simulink model "DrivetrainHevP4_SSC"  (R2021a)
settings: Solver=ode23t  StartTime=0.0  StopTime=10.0  RelTol=1e-3
model workspace (MAT data in the model file):
  Aeff = 0.0314159265359
  Af = 2.27
  Apist_C0 = 0.0314159265359
  Apist_TCC = 0.001
  Bx = 10
  Cd = 0.25
  CoulFr_ShaftIn = 0
  Cx = 1.9
  DensAir = 1.293
  DerFac_C0 = 1
  DerFac_TCC = 1
  Drag_C0 = 0
  Drag_TCC = 0
  Dx = 1
  Eff_Diff = [0.98 0.98]
  Ex = 0.97
  FDrive = 3.32
  FDrive_P4 = 4.1
  FZMAX = 6570
  FZMIN = 0
  G = [0 1 2 3 4 5 6]
  G_o = 1
  Iyy = 0.8
  Iyy_Whl = 0.8
  JCa_Diff = 0.001
  JEng = 0.01
  JMot = 0.21
  JPl_Diff = 0.001
  JShIn = 1e-05
  JShOut = 0.15
  Jd = 0.025
  Ji = 0.21
  Jin_Cltch = 0.2
  Jout = [0.009 0.01 0.01 0.01 0.01 0.01 0.01]
  Jout_Cltch = 0.01
  Jt = 0.01
  Jw1 = 0.01
  Jw2 = 0.01
  K_c = 10000
  KinFr_C0 = 0.4
  KinFr_TCC = 0.3
  Lrel = 0.15
  Mass = 1623
  N = [0.001 4.212 2.637 1.8 1.386 1 0.772]
  NF = 2
  NR = 2
  N_P0 = 3
  Ndiff = 3.32
  Ndiff_P4 = 4.1
  Ndisk = 1
  Neff_C0 = 1
  Neff_TCC = 6
  PEng_C0 = 30000
  PEng_TCC = 100
  Pabs = 101325
  Press = 300000
  PwrThr_Diff = [0.001 0.001]
  RatFr_ShaftIn = 1.1
  Re = 0.327
  Reff = 0.11
  Reff_C0 = 0.11
  Reff_TCC = 130
  Rm = 0.15
  SprStff_ShaftIn = 10000
  StatFr_C0 = 0.45
  StatFr_TCC = 0.35
  T = 273
  Temp_bpts = [313 358]
  Trq_bpts = [25 50 75 100 150 200 250]
  UNLOADED_RADIUS = 0.336
  VXLOW = 2
  VisFr_Diff = [0.001 0.001]
  ViscFr_ShaftIn = 400
  aMy = 0.01
  a_CG = 1.09
  alphaMy = 0
  b : Simulink.Parameter (value not decoded)
  bMy = 0
  b_CG = 1.7
  bd = 0.001
  betaMy = 1
  bi = 0.001
  bin_Cltch = 0.003
  bout = [0.003 0.003 0.003 0.003 0.003 0.003 0.003]
  bout_Cltch = 0.003
  br = 0.001
  bt = 0.001
  bw1 = 0.001
  bw2 = 0.001
  cGain = 100000
  cMy = 0
  disk_abore = 0.05
  domega_o = 0
  eta = [0.95 0.95 0.95 0.95 0.95 0.95 0.95]
  eta_diff = 0.98
  eta_tbl = [1 1 1 1 1 1 1 1 1 1 1 1 ... (1078 elements, 7x11x7x2)]
  g = 9.81
  h = 0.5
  k : Simulink.Parameter (value not decoded)
  kappamax = 1.5
  ki_c = 100000
  lam_x = 1
  mu_kinetic = 0.35
  mu_static = 0.45
  muk = 0.4
  mus = 0.45
  num_pads = 2
  omega_bpts = [500.383141081 749.619781963 1002.67614148 1250.9578527 1499.23956393 1747.52127515 1995.80298637 2501.9157054 2998.47912785 4001.15526933 5003.83141081]
  omega_c : Simulink.Parameter (value not decoded)
  omega_o = 0
  omegai_o = 0
  omegal = 94.2477796077
  omegao = 0
  omegat_o = 0
  omegau = 83.7758040957
  omegaw1o = 0
  omegaw2o = 0
  p0 = 10000000
  phi = [0 0.5 0.6 0.7 0.8 0.87 0.92 0.94 0.96 0.97]
  phi_new = [0 0.5 0.6 0.7 0.8 0.87 0.92 0.94 0.96 0.97 0.99 1.02 ... (16 elements, 1x16)]
  philu = 0.85
  press = 700000
  psi = [12.2938 12.8588 13.1452 13.6285 14.6163 16.2675 19.3503 22.1046 29.9986 50]
  psi_new = [12.2938 12.8588 13.1452 13.6285 14.6163 16.2675 19.3503 22.1046 29.9986 50 48 41.76 ... (16 elements, 1x16)]
  tauC = 0.25
  tauTC = 0.1
  tau_s = 0.1
  theta_o = 0
  wc = 10
  win_o = 0
  wout_o = 0
  x_o = 0
  xdot_o = 0
  zeta = [2.232 1.5462 1.4058 1.2746 1.1528 1.0732 1.0192 0.9983 0.9983 0.9983]
  zeta_new = [2.232 1.5462 1.4058 1.2746 1.1528 1.0732 1.0192 0.9983 0.9983 0.9983 0.979797979798 1.04382929642 ... (16 elements, 1x16)]
libraries: fl_lib x28, sdl_lib x23, nesl_utility x21, simulink x6
(part 2 of 2)

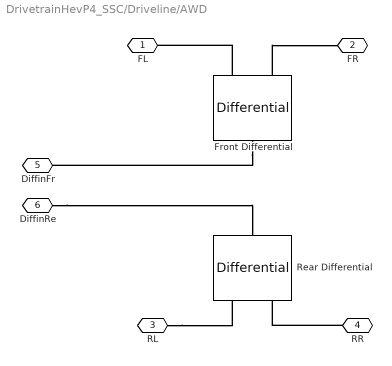
== system DrivetrainHevP4_SSC/Driveline/AWD ==
  Front Differential : sdl_lib/Gears/Differential  driveshaft_location=2  cd_ratio=FDrive  friction_model=2  mu_visc=VisFr_Diff N*m/(rad/s)  efficiency=Eff_Diff  temperature_TLU=[ 280 300 320 ] K  efficiency_ss_TLU=[ 0.95 0.9 0.85 ]  efficiency_cd_TLU=[ 0.95 0.9 0.85 ]  pwr_thr=PwrThr_Diff W  thermal_mass=50 J/K  T_init=300 K  model_inertia=1  carrier_inertia=JCa_Diff kg*m^2  planet_inertia=JPl_Diff kg*m^2
      settings: SourceProductBaseCode=LD
  Rear Differential : sdl_lib/Gears/Differential  driveshaft_location=sdl.enum.differential_orientation.right  cd_ratio=FDrive_P4  friction_model=sdl.enum.gear_friction.constant  mu_visc=VisFr_Diff N*m/(rad/s)  efficiency=Eff_Diff  temperature_TLU=[ 280 300 320 ] K  efficiency_ss_TLU=[ 0.95 0.9 0.85 ]  efficiency_cd_TLU=[ 0.95 0.9 0.85 ]  pwr_thr=PwrThr_Diff W  thermal_mass=50 J/K  T_init=300 K  model_inertia=simscape.enum.onoff.on  carrier_inertia=JCa_Diff kg*m^2  planet_inertia=JPl_Diff kg*m^2
      settings: SourceProductBaseCode=LD
  FL : PMIOPort  Side=Left
  FR : PMIOPort  Port=2  Side=Right
  RL : PMIOPort  Port=3  Side=Left
  RR : PMIOPort  Port=4  Side=Right
  DiffinFr : PMIOPort  Port=5  Side=Left
  DiffinRe : PMIOPort  Port=6  Side=Right
  connections:
  Front Differential/LConn1 -- DiffinFr/RConn1
  Front Differential/RConn1 -- FL/RConn1
  RR/RConn1 -- Rear Differential/RConn2
  RL/RConn1 -- Rear Differential/RConn1
  Front Differential/RConn2 -- FR/RConn1
  DiffinRe/RConn1 -- Rear Differential/LConn1

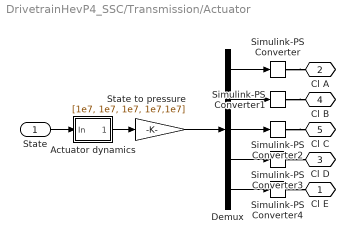
== system DrivetrainHevP4_SSC/Transmission/Actuator ==
  State : Inport
  Actuator dynamics : Subsystem  mask(First-order lag supporting vector signals){b=[1 1 1 1 1]*0.01, x_initial=1}
      mask prompts: b "Filter time constant"; x_initial "Initial output"
      mask help: Models a lag of the form 1/(b*s+1) where s is the Laplace operator.
  Demux : Demux  Outputs=5
  Simulink-PS Converter{,1..4} (5 alike) : nesl_utility/Simulink-PS Converter  PhysicalDomain=network_engine_domain  SubClassName=ps_input  LeftPortType=input  RightPortType=output  PseudoPeriodic=off  Frequencies=[]  NoiseDistribution=none  NoiseParameters=[]  Unit=1  AffineConversion=off  FilteringAndDerivatives=zero  SimscapeFilterOrder=1  InputFilterTimeConstant=0.001  UdotUserProvided=1
      settings: SourceProductBaseCode=PW,SS
  State to pressure : Gain  Gain=[1e7, 1e7, 1e7, 1e7,1e7]
  Cl E : PMIOPort  Side=Right
  Cl A : PMIOPort  Port=2  Side=Right
  Cl D : PMIOPort  Port=3  Side=Right
  Cl B : PMIOPort  Port=4  Side=Right
  Cl C : PMIOPort  Port=5  Side=Right
  wires:
  Demux/3 -> Simulink-PS Converter2/1
  Demux/5 -> Simulink-PS Converter4/1
  State to pressure/1 -> Demux/1
  Demux/4 -> Simulink-PS Converter3/1
  Demux/2 -> Simulink-PS Converter1/1
  Demux/1 -> Simulink-PS Converter/1
  Actuator dynamics/1(Out) -> State to pressure/1
  State/1 -> Actuator dynamics/1(In)
  connections:
  Simulink-PS Converter4/RConn1 -- Cl E/RConn1
  Simulink-PS Converter3/RConn1 -- Cl D/RConn1
  Simulink-PS Converter2/RConn1 -- Cl C/RConn1
  Simulink-PS Converter/RConn1 -- Cl A/RConn1
  Simulink-PS Converter1/RConn1 -- Cl B/RConn1

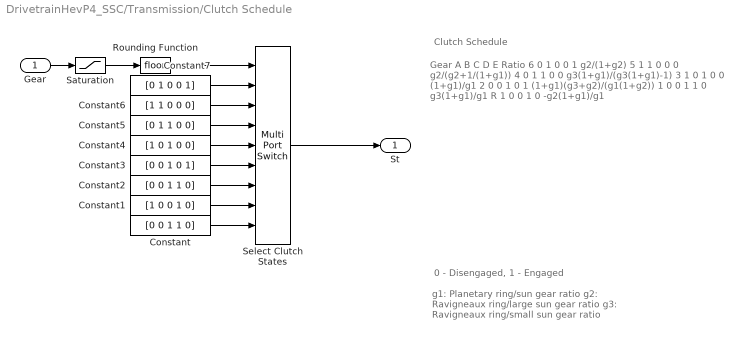
== system DrivetrainHevP4_SSC/Transmission/Clutch Schedule ==
  note: Gear
      | A
      | B
      | C
      | D
      | E
      | Ratio
      |
      | 6
      | 0
      | 1
      | 0
      | 0
      | 1
      | g2/(1+g2)
      |
      | 5
      | 1
      | 1
      | 0
      | 0
      | 0
      | g2/(g2+1/(1+g1))
      |
      | 4
      | 0
      | 1
      | 1
      | 0
      | 0
      | g3(1+g1)/(g3(1+g1)-1)
      |
      | 3
      | 1
      | 0
      | 1
      | 0
      | 0
      | (1+g1)/g1
      |
      | 2
      | 0
      | 0
      | 1
      | 0
      | 1
      | (1+g1)(g3+g2)/(g1(1+g2))
      |
      | 1
      | 0
      | 0
      | 1
      | 1
      | 0
      | g3(1+g1)/g1
      |
      | R
      | 1
      | 0
      | 0
      | 1
      | 0
      | -g2(1+g1)/g1
  note: g1: Planetary ring/sun gear ratio
      | g2: Ravigneaux ring/large sun gear ratio
      | g3: Ravigneaux ring/small sun gear ratio
  note: 0 - Disengaged, 1 - Engaged
  note: Clutch Schedule
  Gear : Inport
  Constant : Constant  Value=[0 0 1 1 0]
  Constant1 : Constant  Value=[1 0 0 1 0]
  Constant2 : Constant  Value=[0 0 1 1 0]
  Constant3 : Constant  Value=[0 0 1 0 1]
  Constant4 : Constant  Value=[1 0 1 0 0]
  Constant5 : Constant  Value=[0 1 1 0 0]
  Constant6 : Constant  Value=[1 1 0 0 0]
  Constant7 : Constant  Value=[0 1 0 0 1]  VectorParams1D=off
  Rounding Function : Rounding
  Saturation : Saturate  UpperLimit=6  LowerLimit=-1  ZeroCross=off
  Select Clutch States : MultiPortSwitch  DataPortOrder=Specify indices  DataPortIndices={6,5,4,3,2,1,-1,0}  DiagnosticForDefault=None
  St : Outport  VectorParamsAs1DForOutWhenUnconnected=off
  wires:
  Select Clutch States/1 -> St/1
  Gear/1 -> Saturation/1
  Constant/1 -> Select Clutch States/9
  Saturation/1 -> Rounding Function/1
  Rounding Function/1 -> Select Clutch States/1
  Constant1/1 -> Select Clutch States/8
  Constant2/1 -> Select Clutch States/7
  Constant3/1 -> Select Clutch States/6
  Constant4/1 -> Select Clutch States/5
  Constant5/1 -> Select Clutch States/4
  Constant6/1 -> Select Clutch States/3
  Constant7/1 -> Select Clutch States/2

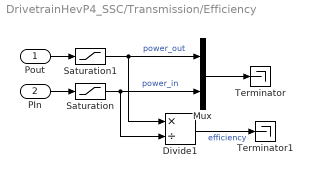
== system DrivetrainHevP4_SSC/Transmission/Efficiency ==
  Pout : Inport
  PIn : Inport  Port=2
  Divide1 : Product  Inputs=*/
  Mux : Mux  Inputs=2
  Saturation : Saturate  UpperLimit=100  LowerLimit=0.1  ZeroCross=off
  Saturation1 : Saturate  UpperLimit=100  LowerLimit=-100  ZeroCross=off
  Terminator : Terminator
  Terminator1 : Terminator
  wires:
  Saturation/1 -> Mux/2, Divide1/2  "power_in"
  Saturation1/1 -> Mux/1, Divide1/1  "power_out"
  Divide1/1 -> Terminator1/1  "efficiency"
  Mux/1 -> Terminator/1
  PIn/1 -> Saturation/1
  Pout/1 -> Saturation1/1

== system DrivetrainHevP4_SSC/Transmission/R ==
  Ideal Rotational Motion Sensor : fl_lib/Mechanical/Mechanical Sensors/Ideal Rotational Motion Sensor  wrap_angle=simscape.enum.onoff.off  offset=0 rad
  MRRef Brake C4 : fl_lib/Mechanical/Rotational Elements/Mechanical Rotational Reference
  PS-Simulink Converter : nesl_utility/PS-Simulink Converter  PhysicalDomain=network_engine_domain  SubClassName=ps_output  LeftPortType=input  RightPortType=output  PseudoPeriodic=off  Frequencies=[]  Unit=1  AffineConversion=off
      settings: SourceProductBaseCode=PW,SS
  B : PMIOPort  Side=Left
  tag scope: w_in=global
  wires:
  PS-Simulink Converter/1 -> [w_in]  "win_ssc"
  connections:
  PS-Simulink Converter/LConn1 -- Ideal Rotational Motion Sensor/RConn2
  MRRef Brake C4/LConn1 -- Ideal Rotational Motion Sensor/RConn1
  Ideal Rotational Motion Sensor/LConn1 -- B/RConn1

== system DrivetrainHevP4_SSC/Transmission/R2 ==
  Ideal Rotational Motion Sensor : fl_lib/Mechanical/Mechanical Sensors/Ideal Rotational Motion Sensor  wrap_angle=simscape.enum.onoff.off  offset=0 rad
  MRRef Brake C4 : fl_lib/Mechanical/Rotational Elements/Mechanical Rotational Reference
  PS-Simulink Converter : nesl_utility/PS-Simulink Converter  PhysicalDomain=network_engine_domain  SubClassName=ps_output  LeftPortType=input  RightPortType=output  PseudoPeriodic=off  Frequencies=[]  Unit=1  AffineConversion=off
      settings: SourceProductBaseCode=PW,SS
  B : PMIOPort  Side=Left
  tag scope: w_out=global
  wires:
  PS-Simulink Converter/1 -> [w_out]  "wout_ssc"
  connections:
  Ideal Rotational Motion Sensor/LConn1 -- B/RConn1
  MRRef Brake C4/LConn1 -- Ideal Rotational Motion Sensor/RConn1
  PS-Simulink Converter/LConn1 -- Ideal Rotational Motion Sensor/RConn2

== system DrivetrainHevP4_SSC/Transmission/Actuator/Actuator dynamics ==
  In : Inport
  Gain : Gain  Gain=1./b
  Integrator : Integrator  InitialCondition=[0 0 0 0 0].*b
  Sum : Sum  Inputs=|+-  InputSameDT=on  SaturateOnIntegerOverflow=on  OutDataTypeStr=Inherit: Same as first input
  Out : Outport  VectorParamsAs1DForOutWhenUnconnected=off
  wires:
  Sum/1 -> Integrator/1
  In/1 -> Sum/1
  Integrator/1 -> Gain/1
  Gain/1 -> Sum/2, Out/1
